simulink model "kinSwCtrl_v2_2"  (R2015a)
settings: Solver=ode45  StartTime=0.0  StopTime=t_sim  RelTol=1e-3
InitFcn:
  | set_kinSwCtrl_v2_2;
StopFcn:
  | plot_kinSwCtrl2;
values from neighbouring files (symbols this model uses):
  alpha_0 = 120*pi/180    (= 2.09439510239)    [set_kinSwCtrl_v2.m]    (also in set_kinSwCtrl_v2_2.m)
  alpha_min = 90*pi/180    (= 1.57079632679)    [set_kinSwCtrl_v2.m]    (also in set_kinSwCtrl_v2_2.m = 1.3962634016)
  alpha_tgt = 70*pi/180    (= 1.2217304764)    [set_kinSwCtrl_v2_2.m]
  l_min = 0.7    [set_kinSwCtrl_v2.m]    (also in set_kinSwCtrl_v2_2.m)
  l_tgt = 0.9    [set_kinSwCtrl_v2_2.m]
  v_alpha = (alpha_min-alpha_0)/t_sim    (= -0.523598775598)    [set_kinSwCtrl_v2.m]    (also in set_kinSwCtrl_v2_2.m = -0.436332312999)
libraries: simulink_extras x2, simulink x1
settings Model: Creator=smsong  LastModifiedBy=smsong

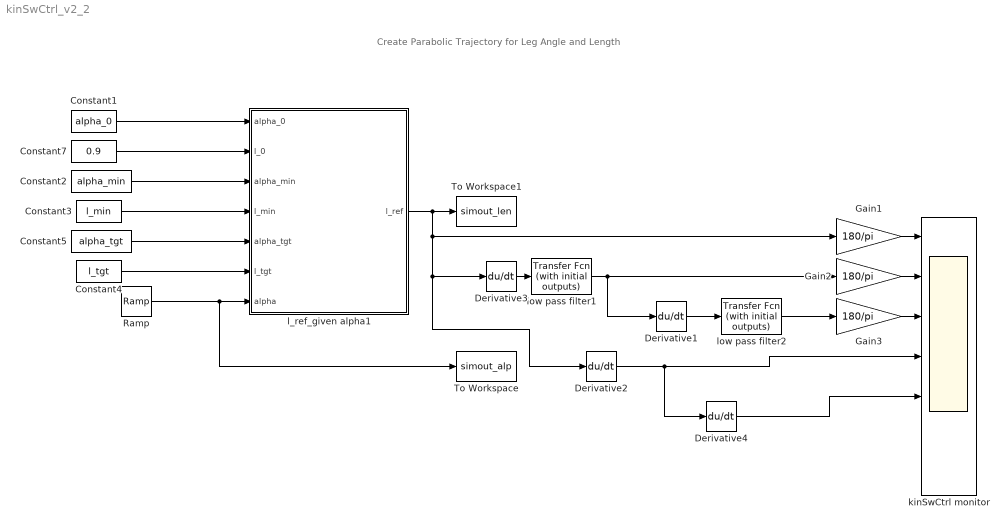
== system kinSwCtrl_v2_2 ==
  note: Create Parabolic
      | Trajectory for Leg Angle and Length
  Constant1 : Constant  Value=alpha_0
  Constant2 : Constant  Value=alpha_min
  Constant3 : Constant  Value=l_min
  Constant4 : Constant  Value=l_tgt
  Constant5 : Constant  Value=alpha_tgt
  Constant7 : Constant  Value=0.9
  Derivative{1..4} (4 alike) : Derivative
  Gain1 : Gain  Gain=180/pi
  Gain2 : Gain  Gain=180/pi
  Gain3 : Gain  Gain=180/pi
  Ramp : simulink/Sources/Ramp  slope=v_alpha  start=0  X0=alpha_0
  To Workspace : ToWorkspace  VariableName=simout_alp  SaveFormat=Structure With Time  SampleTime=-1
  To Workspace1 : ToWorkspace  VariableName=simout_len  SaveFormat=Structure With Time  SampleTime=-1
  kinSwCtrl monitor : Scope  NumInputPorts=7
      settings: YMin=-0.1~-0.1~-0.1~80~-400~-5~-5  YMax=1.1~1.1~1.1~150~300~5~5  SaveName=ScopeData13
  l_ref_given alpha1 : Subsystem
  low pass filter1 : simulink_extras/Additional Linear/Transfer Fcn (with initial outputs)  N=[1]  D="[.5  1]"  Y0=0  U0=0
      settings: AttributesFormatString=pre-activation: %<Y0>
  low pass filter2 : simulink_extras/Additional Linear/Transfer Fcn (with initial outputs)  N=[1]  D="[.5  1]"  Y0=0  U0=0
      settings: AttributesFormatString=pre-activation: %<Y0>
  wires:
  Constant7/1 -> l_ref_given alpha1/2(l_0)
  Constant1/1 -> l_ref_given alpha1/1(alpha_0)
  Constant2/1 -> l_ref_given alpha1/3(alpha_min)
  Constant3/1 -> l_ref_given alpha1/4(l_min)
  Constant4/1 -> l_ref_given alpha1/6(l_tgt)
  Constant5/1 -> l_ref_given alpha1/5(alpha_tgt)
  Ramp/1 -> To Workspace/1, l_ref_given alpha1/7(alpha)
  Derivative3/1 -> low pass filter1/1
  Derivative1/1 -> low pass filter2/1
  l_ref_given alpha1/1(l_ref) -> Derivative3/1, Derivative2/1, Gain1/1, To Workspace1/1
  Gain1/1 -> kinSwCtrl monitor/1
  Gain2/1 -> kinSwCtrl monitor/2
  Gain3/1 -> kinSwCtrl monitor/3
  low pass filter1/1 -> Derivative1/1, Gain2/1
  Derivative2/1 -> Derivative4/1, kinSwCtrl monitor/4
  Derivative4/1 -> kinSwCtrl monitor/5
  low pass filter2/1 -> Gain3/1

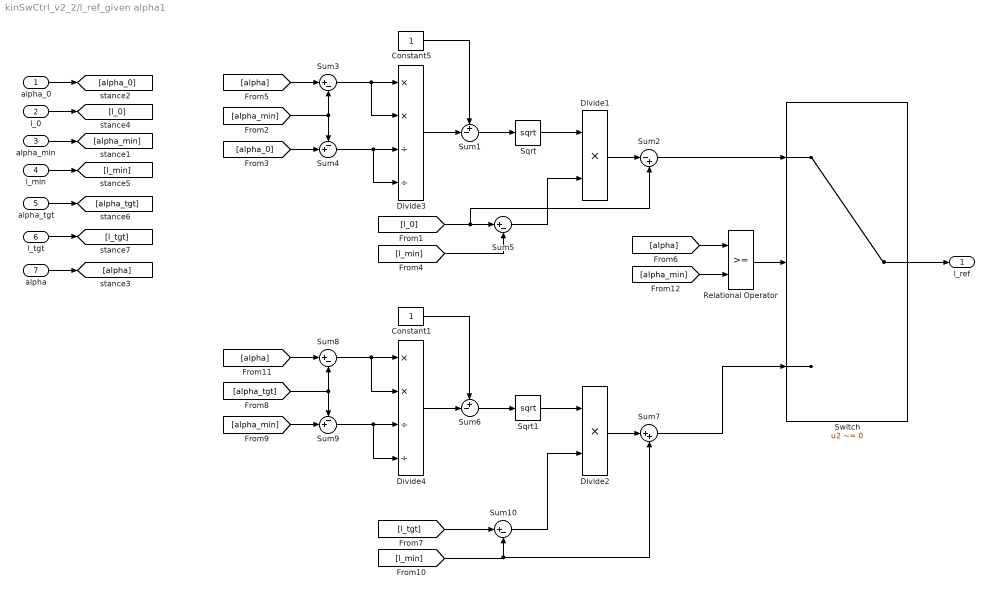
== system kinSwCtrl_v2_2/l_ref_given alpha1 ==
  alpha_0 : Inport
  l_0 : Inport  Port=2
  alpha_min : Inport  Port=3
  l_min : Inport  Port=4
  alpha_tgt : Inport  Port=5
  l_tgt : Inport  Port=6
  alpha : Inport  Port=7
  Constant1 : Constant
  Constant5 : Constant
  Divide1 : Product
  Divide2 : Product
  Divide3 : Product  Inputs=**//
  Divide4 : Product  Inputs=**//
  Relational Operator : RelationalOperator  OutDataTypeStr=boolean
  Sqrt : Sqrt  SaturateOnIntegerOverflow=on
  Sqrt1 : Sqrt  SaturateOnIntegerOverflow=on
  Sum1 : Sum  Inputs=+-|
  Sum{3,5,8,10} (4 alike) : Sum  Inputs=|+-
  Sum2 : Sum  Inputs=|-+
  Sum4 : Sum  Inputs=-+|
  Sum6 : Sum  Inputs=+-|
  Sum7 : Sum  Inputs=|++
  Sum9 : Sum  Inputs=-+|
  Switch : Switch  Criteria=u2 ~= 0
  l_ref : Outport
  wires:
  alpha/1 -> [alpha]
  alpha_min/1 -> [alpha_min]
  alpha_0/1 -> [alpha_0]
  l_0/1 -> [l_0]
  l_min/1 -> [l_min]
  Constant5/1 -> Sum1/1
  [alpha_min] -> Sum3/2, Sum4/1
  [alpha] -> Sum3/1
  Sum3/1 -> Divide3/2, Divide3/1
  [alpha_0] -> Sum4/2
  Sum4/1 -> Divide3/4, Divide3/3
  Divide3/1 -> Sum1/2
  Sum1/1 -> Sqrt/1
  Sqrt/1 -> Divide1/1
  [l_min] -> Sum5/2
  Sum5/1 -> Divide1/2
  Divide1/1 -> Sum2/1
  Sum2/1 -> Switch/1
  Switch/1 -> l_ref/1
  [l_0] -> Sum2/2, Sum5/1
  Constant1/1 -> Sum6/1
  [alpha_tgt] -> Sum8/2, Sum9/1
  [alpha] -> Sum8/1
  Sum8/1 -> Divide4/2, Divide4/1
  [alpha_min] -> Sum9/2
  Sum9/1 -> Divide4/4, Divide4/3
  Divide4/1 -> Sum6/2
  Sum6/1 -> Sqrt1/1
  Sqrt1/1 -> Divide2/1
  [l_min] -> Sum7/2, Sum10/2
  Sum10/1 -> Divide2/2
  Divide2/1 -> Sum7/1
  Sum7/1 -> Switch/3
  [l_tgt] -> Sum10/1
  alpha_tgt/1 -> [alpha_tgt]
  l_tgt/1 -> [l_tgt]
  Relational Operator/1 -> Switch/2
  [alpha] -> Relational Operator/1
  [alpha_min] -> Relational Operator/2
